simulink model "OBServer"  (Simulink 10.3)
settings: Solver=ode45  StartTime=0.0  StopTime=1000  RelTol=1e-3  EnableMultiTasking=on
values from neighbouring files (symbols this model uses):
  D = [dxd+bb1;dyd+bb2]    [alfuv.m]    (also in constant.m = diag([d11,d22,d33]))
  K01 = diag([1,1,1])    [constant.m]
  M = diag([m11,m22,m33])    [constant.m]
settings Model: Creator=Administrator  LastModifiedBy=1179956468
settings DataIOCC: LimitDataPoints=on
settings DebuggingCC: SolverPrmCheckMsg=warning
settings GRTTargetCC: CombineOutputUpdateFcns=on  GRTInterface=off

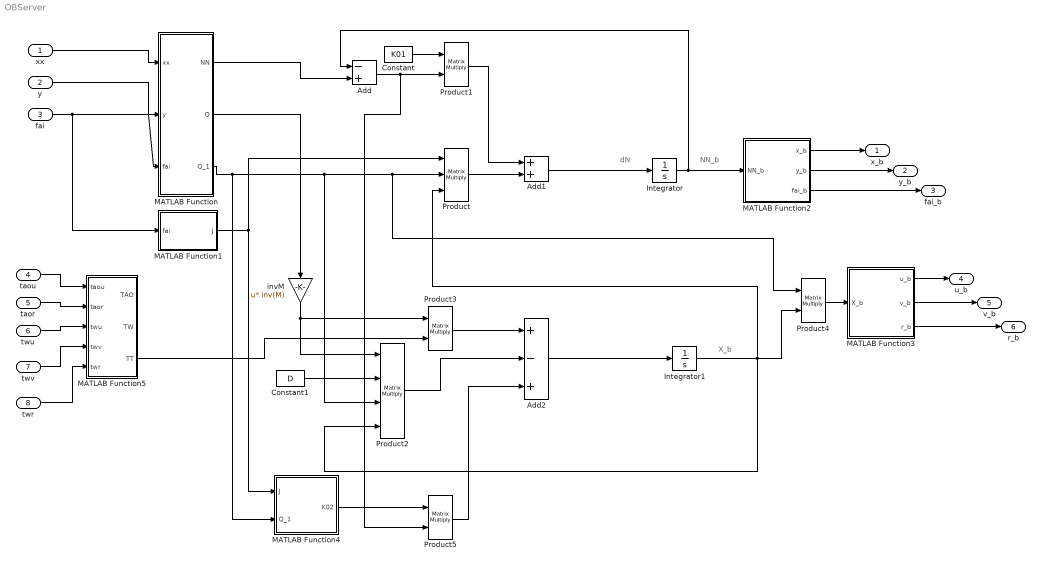
== system OBServer ==
  note: dN
  note: NN_b
  note: X_b
  xx : Inport
  y : Inport  Port=2
  fai : Inport  Port=3
  taou : Inport  Port=4
  taor : Inport  Port=5
  twu : Inport  Port=6
  twv : Inport  Port=7
  twr : Inport  Port=8
  Add : Sum  Inputs=-+
  Add1 : Sum
  Add2 : Sum  Inputs=+-+
  Constant : Constant  Value=K01
  Constant1 : Constant  Value=D
  Integrator : Integrator
  Integrator1 : Integrator
  MATLAB Function : MATLAB Function  TreatAsAtomicUnit=on
  MATLAB Function1 : MATLAB Function  TreatAsAtomicUnit=on
  MATLAB Function2 : MATLAB Function  TreatAsAtomicUnit=on
  MATLAB Function3 : MATLAB Function  TreatAsAtomicUnit=on
  MATLAB Function4 : MATLAB Function  TreatAsAtomicUnit=on
  MATLAB Function5 : MATLAB Function  TreatAsAtomicUnit=on
  Product : Product  Inputs=3  Multiplication=Matrix(*)  RndMeth=Zero
  Product{1,3..5} (4 alike) : Product  Multiplication=Matrix(*)  RndMeth=Zero
  Product2 : Product  Inputs=4  Multiplication=Matrix(*)  RndMeth=Zero
  invM : Gain  Gain=inv(M)  Multiplication=Matrix(u*K)
  x_b : Outport
  y_b : Outport  Port=2
  fai_b : Outport  Port=3
  u_b : Outport  Port=4
  v_b : Outport  Port=5
  r_b : Outport  Port=6
  wires:
  MATLAB Function5/3(TT) -> Product3/2
  twr/1 -> MATLAB Function5/5(twr)
  twv/1 -> MATLAB Function5/4(twv)
  twu/1 -> MATLAB Function5/3(twu)
  taor/1 -> MATLAB Function5/2(taor)
  taou/1 -> MATLAB Function5/1(taou)
  Product5/1 -> Add2/3
  MATLAB Function4/1(K02) -> Product5/1
  xx/1 -> MATLAB Function/1(xx)
  y/1 -> MATLAB Function/2(y)
  fai/1 -> MATLAB Function/3(fai), MATLAB Function1/1(fai)
  Add1/1 -> Integrator/1
  Integrator1/1 -> Product/3, Product2/4, Product4/2
  Product/1 -> Add1/2
  Integrator/1 -> Add/1, MATLAB Function2/1(NN_b)
  Product1/1 -> Add1/1
  MATLAB Function/3(Q_1) -> Product2/3, Product/2, Product4/1, MATLAB Function4/2(Q_1)
  MATLAB Function1/1(J) -> Product/1, MATLAB Function4/1(J)
  MATLAB Function/1(NN) -> Add/2
  Add/1 -> Product1/2, Product5/2
  Constant/1 -> Product1/1
  MATLAB Function/2(Q) -> invM/1
  invM/1 -> Product2/1, Product3/1
  Constant1/1 -> Product2/2
  Product3/1 -> Add2/1
  Product2/1 -> Add2/2
  Add2/1 -> Integrator1/1
  MATLAB Function2/1(x_b) -> x_b/1
  MATLAB Function2/2(y_b) -> y_b/1
  MATLAB Function2/3(fai_b) -> fai_b/1
  MATLAB Function3/1(u_b) -> u_b/1
  MATLAB Function3/2(v_b) -> v_b/1
  MATLAB Function3/3(r_b) -> r_b/1
  Product4/1 -> MATLAB Function3/1(X_b)

== matlab function MATLAB Function1 ==
  data: fai input double; J output double
function J = fcn(fai)
%#codegen

J=[cos(fai) -sin(fai) 0;
    sin(fai) cos(fai) 0;
    0 0 1];

== matlab function MATLAB Function ==
  data: xx input double; y input double; fai input double; NN output double; Q output double; Q_1 output double
function [NN,Q,Q_1] = fcn(xx,y,fai)
%#codegen
m11=1.2*10^5;m22=1.779*10^5;m33=6.36*10^7;
d11=2.15*10^4;d22=1.47*10^5;d33=8.02*10^6;
NN=[xx;y;fai];
% TAO=[taou;0;taor];
alfa=m22/m11;
beta=m11/m33;
gama=m22/m33;
f=xx*sin(fai)-y*cos(fai);
h=xx*cos(fai)+y*sin(fai);
Q =[cos(fai) -alfa*sin(fai) 0;sin(fai) alfa*cos(fai) 0;f*beta h*gama 1];
Q_1=inv(Q);

== matlab function MATLAB Function2 ==
  data: NN_b input double; x_b output double; y_b output double; fai_b output double
function [x_b,y_b,fai_b] = fcn(NN_b)
%#codegen

x_b=[1 0 0]*NN_b;
y_b=[0 1 0]*NN_b;
fai_b=[0 0 1]*NN_b;

== matlab function MATLAB Function3 ==
  data: X_b input double; u_b output double; v_b output double; r_b output double
function [u_b,v_b,r_b] = fcn(X_b)
%#codegen

u_b=[1 0 0]*X_b;
v_b=[0 1 0]*X_b;
r_b=[0 0 1]*X_b;

== matlab function MATLAB Function4 ==
  data: J input double; K02 output double; Q_1 input double
function K02= fcn(J,Q_1)
%#codegen

K02=(J*Q_1)';

== matlab function MATLAB Function5 ==
  data: taou input double; TAO output double; taor input double; twu input double; twv input double; twr input double; TW output double; TT output double
function [TAO,TW,TT]= fcn(taou,taor,twu,twv,twr)
%#codegen
TAO=[taou;0;taor];
TW=[twu;twv;twr];
TT=TAO+TW;
